simulink model "ThdynConvTest"  (R2013a)
settings: Solver=ode4  StartTime=0  StopTime=1000  FixedStep=1e-3  RelTol=1e-5  AbsTol=1e-5
values from neighbouring files (symbols this model uses):
  B = [B1;B2]    [GensetRespOptimiztion.m]    (also in GensetRespOptimiztionTorstein.m; Init8RTFLEX68D.m = 0.68; init_MVM.m = 0.127)
  F = interp1(tArray,FCyl,t)    [NOxProcessGUI.m]    (also in ThdynCVTestScript.m = 0.3; ThdynTest.m = 0)
  FExh0 = 0    [Init8RTFLEX68D.m]
  fs = 0.0683    [Init8RTFLEX68D.m]    (also in NOxProcessGUI.m = varargin{2}; initHybrid.m; initMV.m; init_MVM.m = 0.0682925799315)
  FScav0 = 0    [Init8RTFLEX68D.m]
  p = diff(T_temp,dtheta)    [ICModelCrankMechanism.m]    (also in NOxProcessGUI.m = interp1(tArray,pCyl,t); ThdynCVTestScript.m = 150000; ThdynTest.m = 100000; Untitled2.m = 0:0.01:1)
  pExh0 = pExhRef(caseInit)    [Init8RTFLEX68D.m]
  pScav0 = pScavRef(caseInit)    [Init8RTFLEX68D.m]
  RPM0 = simin(1,2)    [Init8RTFLEX68D.m]
  stroke = 2.72    [Init8RTFLEX68D.m]
  T = 0.5*mP*dxP^2 + 0.5*mCR1*dxCR1^2 + 0.5*jCR1*dphi_sqr      + 0.5*jCR2*diff(theta,t)^2    [ICModelCrankMechanism.m]    (also in NOxProcessGUI.m = interp1(tArray,TCyl,t); ThdynCVTestScript.m = 320; ThdynTest.m = 300)
  TExh0 = TExhRef(caseInit)    [Init8RTFLEX68D.m]
  TScav0 = TScavRef(caseInit)    [Init8RTFLEX68D.m]
  VCV = 1.2    [ThdynCVTestScript.m]    (also in ThdynTest.m = 1)
libraries: EngineSysteSubmodel x1
settings Model: Creator=yum  LastModifiedBy=yum
settings DataIOCC: SaveFormat=StructureWithTime  ReturnWorkspaceOutputs=on

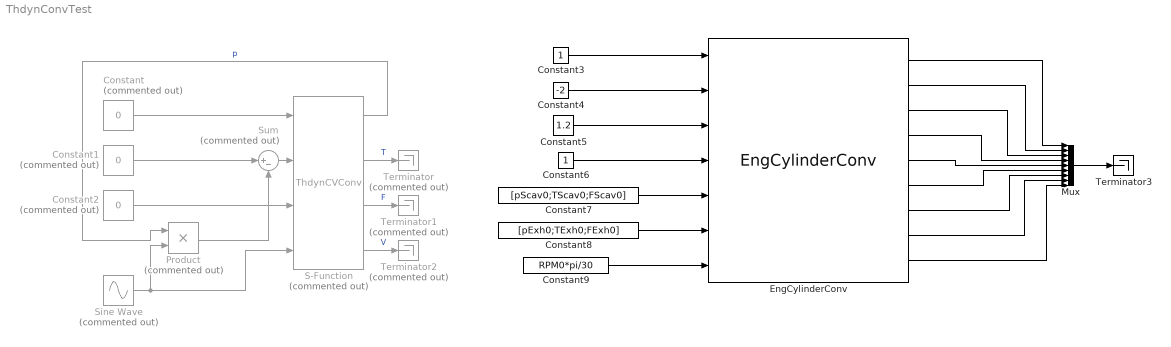
== system ThdynConvTest ==
  Constant : Constant  Commented=on  Value=0
  Constant1 : Constant  Commented=on  Value=0
  Constant2 : Constant  Commented=on  Value=0
  Constant3 : Constant
  Constant4 : Constant  Value=-2
  Constant5 : Constant  Value=1.2
  Constant6 : Constant
  Constant7 : Constant  Value=[pScav0;TScav0;FScav0]
  Constant8 : Constant  Value=[pExh0;TExh0;FExh0]
  Constant9 : Constant  Value=RPM0*pi/30
  EngCylinderConv : EngineSysteSubmodel/EngCylinderConv  fs=fs  nStroke=2  hn=hn  nCyl=nCyl  iCyl=1  B=B  stroke=stroke  lambdaCrank=lambdaCrank  aCrank=stroke/2  X=X  Y=Y  r=r  nPort=nPort  liftMax=liftMax  Dv=Dv  beta=beta  w=w  Dp=Dp  Ds=Ds  cAVVUpRef=cAVVUpRef  cAVVDownRef=cAVVDownRef  liftUpRef=liftUpRef  liftDownRef=liftDownRef  cAStartRef=cAStartRef  dCALiftUp=dCALiftUp  dCALiftDown=dCALiftDown  dCALiftTopRef=dCALiftTopRef  mCp=mCp  cCylHT=cCylHT  cAlpha=cAlpha  mqfCycMax=mqfCycMax  wiebePara=wiebePara  phi0=phi0  p0=0  T0=0  F0=0  V0=0  phi0A=phi0  p0A=pCyl0  T0A=TCyl0  F0A=FCyl0  V0A=vCyl0
  Mux : Mux  Inputs=9
  Product : Product  Commented=on
  S-Function : S-Function  Commented=on  FunctionName=ThdynCVConv  Parameters=fs,p,T,F,VCV  EnableBusSupport=off
  Sine Wave : Sin  Commented=on  Amplitude=-0.25*10  Frequency=10  SampleTime=0
  Sum : Sum  Commented=on  Inputs=|+-
  Terminator : Terminator  Commented=on
  Terminator1 : Terminator  Commented=on
  Terminator2 : Terminator  Commented=on
  Terminator3 : Terminator
  wires:
  Constant/1 -> S-Function/1
  Constant1/1 -> Sum/1
  Constant2/1 -> S-Function/3
  S-Function/1 -> Product/1  "p"
  Sine Wave/1 -> S-Function/4, Product/2
  Sum/1 -> S-Function/2
  Product/1 -> Sum/2
  S-Function/2 -> Terminator/1  "T"
  S-Function/3 -> Terminator1/1  "F"
  S-Function/4 -> Terminator2/1  "V"
  Constant3/1 -> EngCylinderConv/1
  Constant4/1 -> EngCylinderConv/2
  Constant5/1 -> EngCylinderConv/3
  Constant6/1 -> EngCylinderConv/4
  Constant7/1 -> EngCylinderConv/5
  Constant8/1 -> EngCylinderConv/6
  Constant9/1 -> EngCylinderConv/7
  EngCylinderConv/1 -> Mux/1
  EngCylinderConv/2 -> Mux/2
  EngCylinderConv/3 -> Mux/3
  EngCylinderConv/4 -> Mux/4
  EngCylinderConv/5 -> Mux/5
  EngCylinderConv/6 -> Mux/6
  EngCylinderConv/7 -> Mux/7
  EngCylinderConv/8 -> Mux/8
  EngCylinderConv/9 -> Mux/9
  Mux/1 -> Terminator3/1
